simulink model "Lab1SimulinkModel"  (R2022b)
settings: Solver=VariableStepAuto  StartTime=0.0  StopTime=0.1  RelTol=1e-3
values from neighbouring files (symbols this model uses):
  J = 1/(3.88e-5)    (= 25773.1958763)    [Lab1_Preparation.m]
  L = 1/(3.39e-3)    (= 294.985250737)    [Lab1_Preparation.m]
  Mu = 1.194e-4    (= 0.0001194)    [Lab1_Preparation.m]
  R = 1.15    [Lab1_Preparation.m]
  r = 0.056    [Lab1_Preparation.m]
settings Model: Creator=manun  LastModifiedBy=manun

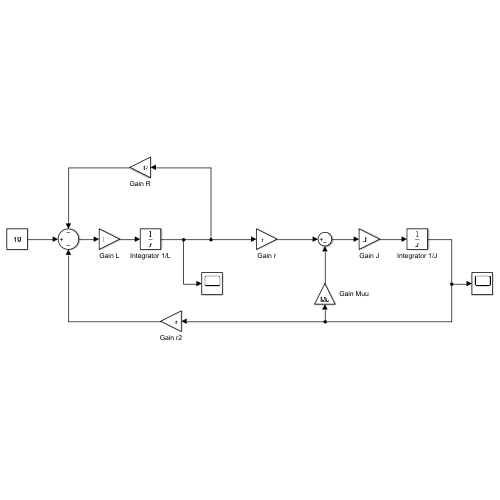
[thumbnail: Simulink's stored preview of the top-level diagram]
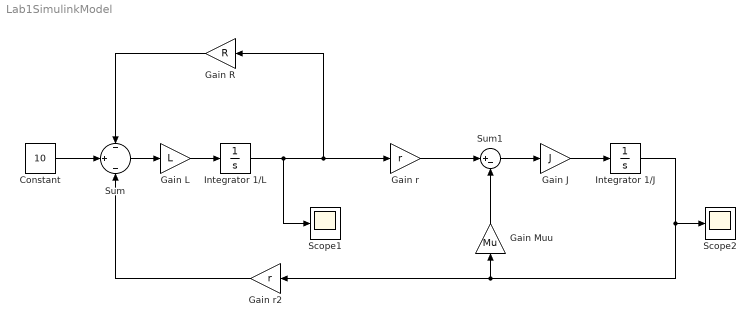
== system Lab1SimulinkModel ==
  Constant : Constant  Value=10
  Gain J : Gain  Gain=J
  Gain L : Gain  Gain=L
  Gain Muu : Gain  Gain=Mu
  Gain R : Gain  Gain=R
  Gain r : Gain  Gain=r
  Gain r2 : Gain  Gain=r
  Integrator 1/J : Integrator
  Integrator 1/L : Integrator
  Scope1 : Scope
  Scope2 : Scope
  Sum : Sum  Inputs=-|+|-
  Sum1 : Sum  Inputs=|+-
  wires:
  Integrator 1/L/1 -> Gain r/1, Gain R/1, Scope1/1
  Gain R/1 -> Sum/1
  Gain r/1 -> Sum1/1
  Sum1/1 -> Gain J/1
  Gain Muu/1 -> Sum1/2
  Integrator 1/J/1 -> Scope2/1, Gain r2/1, Gain Muu/1
  Sum/1 -> Gain L/1
  Constant/1 -> Sum/2
  Gain L/1 -> Integrator 1/L/1
  Gain J/1 -> Integrator 1/J/1
  Gain r2/1 -> Sum/3
